simulink model "Antriebsstrangmodell_V1_4_n5"  (R2019a)
settings: Solver=FixedStepAuto  StartTime=0.0  StopTime=t_Simulation  FixedStep=dt  RelTol=1e-3
values from neighbouring files (symbols this model uses):
  A_Stirn = 2    [SIMULA~1.M]    (also in SIMULA~2.M)
  alpha_Luft = -4e-3    (= -0.004)    [SIMULA~1.M]    (also in SIMULA~2.M)
  alpha_Rotor = alpha_Al    (= 0.004)    [SIMULA~1.M]    (also in SIMULA~2.M)
  alpha_Stator = alpha_Al    (= 0.004)    [SIMULA~1.M]    (also in SIMULA~2.M)
  alpha_Ummag = -0.75e-3    (= -0.00075)    [SIMULA~1.M]    (also in SIMULA~2.M)
  c_W = 0.37    [SIMULA~1.M]    (also in SIMULA~2.M)
  COG_x = 1.4267    [SIMULA~1.M]    (also in SIMULA~2.M)
  COG_z = 0.4572    [SIMULA~1.M]    (also in SIMULA~2.M)
  cp_Luft = 1008.8    [SIMULA~1.M]    (also in SIMULA~2.M)
  e_Fahrzeug = 1.0478    [SIMULA~1.M]    (also in SIMULA~2.M)
  eta_EMaschine_Break_M_EMaschine = flipud(KennfeldMaschine.M(:,1))'    [SIMULA~1.M]    (also in SIMULA~2.M)
  eta_EMaschine_Break_M_EMaschine_reku = -KennfeldMaschine.M(:,1)'    [SIMULA~1.M]    (also in SIMULA~2.M)
  eta_EMaschine_Break_n_EMaschine = KennfeldMaschine.n(end-1,:)    [SIMULA~1.M]    (also in SIMULA~2.M)
  eta_EMaschine_Break_n_EMaschine_reku = KennfeldMaschine.n(end-1,:)    [SIMULA~1.M]    (also in SIMULA~2.M)
  eta_EMaschine_Faktor_Volllast = 0.98    [SIMULA~1.M]    (also in SIMULA~2.M)
  eta_EMaschine_Table = flip(KennfeldMaschine.etages,1)    [SIMULA~1.M]    (also in SIMULA~2.M)
  eta_EMaschine_Table_reku = KennfeldMaschine.etages    [SIMULA~1.M]    (also in SIMULA~2.M)
  eta_Getriebe = 0.96    [SIMULA~1.M]    (also in SIMULA~2.M)
  eta_IA = 0.5    [SIMULA~1.M]    (also in SIMULA~2.M)
  h_WC_pumpoff = Nu_WC*lam_WC/dh_WC    [SIMULA~1.M]    (also in SIMULA~2.M)
  h_WC_pumpon = Nu_WC*lam_WC/dh_WC    [SIMULA~1.M]    (also in SIMULA~2.M)
  i_Getriebe = 5.697    [SIMULA~1.M]    (also in SIMULA~2.M)
  krb_Korrektur = 0.53/10    (= 0.053)    [SIMULA~1.M]    (also in SIMULA~2.M)
  lam_Luft = 0.028592    [SIMULA~1.M]    (also in SIMULA~2.M)
  M_EMaschine_max = zeros(2,numel(eta_EMaschine_Break_n_EMaschine))    [SIMULA~1.M]    (also in SIMULA~2.M)
  m_Fahrzeug = 825    [SIMULA~1.M]    (also in SIMULA~2.M)
  m_Zuladung = 80    [SIMULA~1.M]    (also in SIMULA~2.M)
  nue_Luft = 19.230034390524e-6    (= 1.92300343905e-05)    [SIMULA~1.M]    (also in SIMULA~2.M)
  pump_start_limit = 273.15 + 33    (= 306.15)    [SIMULA~1.M]    (also in SIMULA~2.M)
  r_dynamisch = 0.2774    [SIMULA~1.M]    (also in SIMULA~2.M)
  rho_Luft = 1.2    [SIMULA~1.M]    (also in SIMULA~2.M)
  rho_Luft_EM = 1.0468    [SIMULA~1.M]    (also in SIMULA~2.M)
  share_EMaschine_Ummagnet_reku_Table = ser.gen.share_Ummagnetisierungsverluste    [SIMULA~1.M]    (also in SIMULA~2.M)
  share_EMaschine_Ummagnet_Table = ser.mot.share_Ummagnetisierungsverluste    [SIMULA~1.M]    (also in SIMULA~2.M)
  share_EMaschine_Wicklung_reku_Table = ser.gen.share_Wicklungsverluste    [SIMULA~1.M]    (also in SIMULA~2.M)
  share_EMaschine_Wicklung_Table = ser.mot.share_Wicklungsverluste    [SIMULA~1.M]    (also in SIMULA~2.M)
  share_EMaschine_WirkMech_reku_Table = ser.gen.share_WirkmechVerluste    [SIMULA~1.M]    (also in SIMULA~2.M)
  share_EMaschine_WirkMech_Table = ser.mot.share_WirkmechVerluste    [SIMULA~1.M]    (also in SIMULA~2.M)
  share_EMaschine_WirkZus_reku_Table = ser.gen.share_WirkZusVerl    [SIMULA~1.M]    (also in SIMULA~2.M)
  share_EMaschine_WirkZus_Table = ser.mot.share_WirkZusVerl    [SIMULA~1.M]    (also in SIMULA~2.M)
  T_Entwurf_Rotor = 273.15+20    (= 293.15)    [SIMULA~1.M]    (also in SIMULA~2.M)
  T_Entwurf_Stator = 273.15+20    (= 293.15)    [SIMULA~1.M]    (also in SIMULA~2.M)
  t_Simulation = v_Fahrzeug.Time(end)+1    [SIMULA~1.M]    (also in SIMULA~2.M = v_Fahrzeug.Time(end))
  T_Start_EMaschine = 273.15 + 23    (= 296.15)    [SIMULA~1.M]    (also in SIMULA~2.M)
  v_max = 110    [SIMULA~1.M]    (also in SIMULA~2.M)
  WB = 2.96    [SIMULA~1.M]    (also in SIMULA~2.M)
undefined symbols (not defined in the file or in its folder): A_AGP, A_IA, Anteil_Rotor_Ringe, Anteil_Stator, chi_Lager, D_2a, D_2r, delta, f_R, m_RTO, m_RYO, m_SSL_L, m_STO, m_SYO, m_WH_L, n_dis
libraries: fl_lib x440, nesl_utility x106, SimscapeCustomBlocks_lib x45, simulink x3
(part 4 of 5)

== system Antriebsstrangmodell_V1_4_n5/Antriebsstrang/E-Maschine Thermik/Wärmeübergangskoeffizienten Konvektion Luftspalt und Endcap-Luft ==
  <n_EMaschine [min^-1]> : Inport
  Abs : Abs
  Constant : Constant  Value=D_2a
  Divide : Product  Inputs=**
  Endcap-Luft-Konvektion : Subsystem
  Gain : Gain  Gain=2*pi/60
  Gain1 : Gain  Gain=0.5
  Luftspalt-Konvektion : Subsystem
  HTC_Luftspalt [W*m^-2*K^-1] : Outport
  HTC_fconv_Luftspalt [W*m^-2*K^-1] : Outport  Port=2
  HTC_Innenluft [W*m^-2*K^-1] : Outport  Port=3
  HTC_fconv_Innenluft [W*m^-2*K^-1] : Outport  Port=4
  wires:
  Gain1/1 -> Luftspalt-Konvektion/1(Rotorradius [m]), Divide/1  "Rotorradius [m]"
  <n_EMaschine [min^-1]>/1 -> Abs/1
  Constant/1 -> Gain1/1
  Abs/1 -> Gain/1, Endcap-Luft-Konvektion/1(n_EMaschine [min^-1])
  Gain/1 -> Divide/2
  Divide/1 -> Luftspalt-Konvektion/2(v_Luftspalt [m*s^-1])  "v_Luftspalt [m*s^-1]"
  Luftspalt-Konvektion/1(HTC_Luftspalt [W*m^-2*K^-1]) -> HTC_Luftspalt [W*m^-2*K^-1]/1
  Endcap-Luft-Konvektion/1(HTC_Innenluft [W*m^-2*K^-1]) -> HTC_Innenluft [W*m^-2*K^-1]/1
  Endcap-Luft-Konvektion/2(HTC_fconv_Innenluft [W*m^-2*K^-1]) -> HTC_fconv_Innenluft [W*m^-2*K^-1]/1
  Luftspalt-Konvektion/2(HTC_fconv_Luftspalt [W*m^-2*K^-1]) -> HTC_fconv_Luftspalt [W*m^-2*K^-1]/1

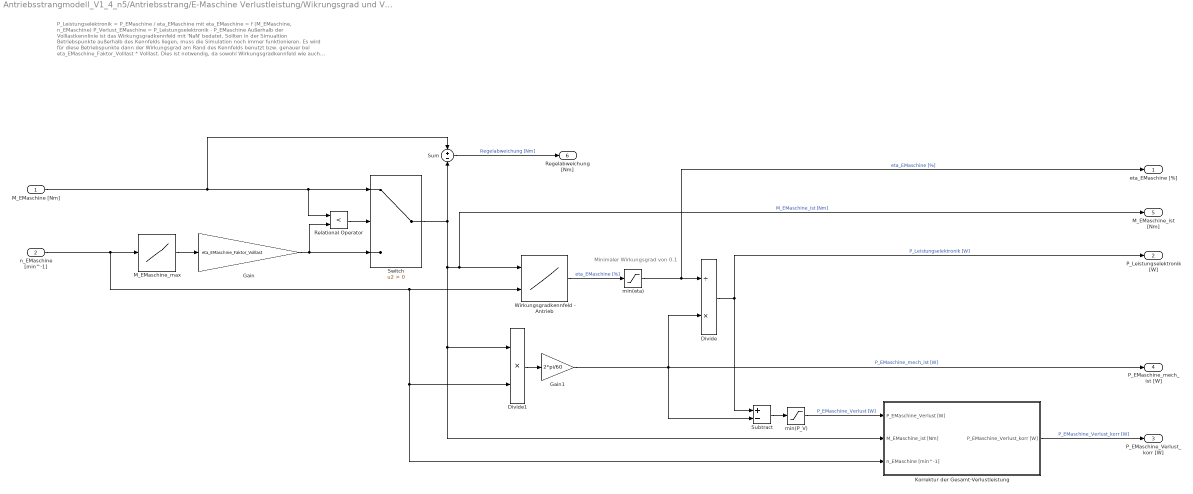
== system Antriebsstrangmodell_V1_4_n5/Antriebsstrang/E-Maschine Verlustleistung/Wikrungsgrad und Verlustleistung - Antrieb ==
  note: Minimaler Wirkungsgrad von 0.1
  note: P_Leistungselektronik = P_EMaschine / eta_EMaschine
      |
      | mit eta_EMaschine = f (M_EMaschine, n_EMaschine)
      |
      | P_Verlust_EMaschine = P_Leistungselektronik - P_EMaschine
      |
      | Außerhalb der Volllastkennlinie ist das Wirkungsgradkennfeld mit 'NaN' bedatet. Sollten in der Simualtion Betriebspunkte außerhalb des Kennfelds liegen, muss die Simulation noch immer funktionieren. Es wird für diese Betriebspunkte dann der Wirkungsgrad am Rand des Kennfelds benutzt bzw. genauer bei eta_EMaschine_Faktor_Volllast * Volllast. Dies ist notwendig, da sowohl Wirkungsgradkennfeld wie auch Lookup Table nicht stetig sind und somit zwischen Stützstellen interpolieren müssen. Dies kann dazu führen, dass ein Wert, der auf der Volllastlinie sitzt, in 'NaN' im Wirkungsgradkennfeld resultiert. Um dies zu vermeiden, wird mit eta_EMaschine_Faktor_Volllast * Volllast gerechnet, wenn Betriebspunkte außerhalb des Kennfelds liegen, um 'NaN' Wirkungsgrade zu vermeiden. eta_EMaschine_Faktor_Volllast ist stark abh. von der Güte (Abstand der Stützstellen) des Wirkungsgradkennfeldes.
  M_EMaschine [Nm] : Inport
  n_EMaschine [min^-1] : Inport  Port=2
  Divide : Product  Inputs=/*
  Divide1 : Product  Inputs=**
  Gain : Gain  Gain=eta_EMaschine_Faktor_Volllast
  Gain1 : Gain  Gain=2*pi/60
  Korrektur der Gesamt-Verlustleistung : Subsystem
  M_EMaschine_max : Lookup_n-D  NumberOfTableDimensions=1  BreakpointsForDimension1=M_EMaschine_max(1,:)  BeginIndexSearchUsingPreviousIndexResult=on  Table=M_EMaschine_max(2,:)  ExtrapMethod=Clip  UseLastTableValue=on  InternalRulePriority=Speed  RndMeth=Simplest  InputSameDT=on
  Relational Operator : RelationalOperator  Operator=<  OutDataTypeStr=boolean  RndMeth=Simplest
  Subtract : Sum  Inputs=+-
  Sum : Sum  Inputs=+-
  Switch : Switch  Criteria=u2 > Threshold
  Wirkungsgradkennfeld - Antrieb : Lookup_n-D  BreakpointsForDimension1=eta_EMaschine_Break_M_EMaschine  BreakpointsForDimension2=eta_EMaschine_Break_n_EMaschine  BeginIndexSearchUsingPreviousIndexResult=on  Table=eta_EMaschine_Table  ExtrapMethod=Clip  UseLastTableValue=on  InternalRulePriority=Speed  RndMeth=Simplest  InputSameDT=on
  min(P_V) : Saturate  UpperLimit=inf  LowerLimit=0
  min(eta) : Saturate  UpperLimit=inf  LowerLimit=0.1
  eta_EMaschine [%] : Outport
  P_Leistungselektronik [W] : Outport  Port=2
  P_EMaschine_Verlust_korr [W] : Outport  Port=3
  P_EMaschine_mech_ist [W] : Outport  Port=4
  M_EMaschine_ist [Nm] : Outport  Port=5
  Regelabweichung [Nm] : Outport  Port=6
  wires:
  Relational Operator/1 -> Switch/2
  Switch/1 -> M_EMaschine_ist [Nm]/1, Wirkungsgradkennfeld - Antrieb/1, Korrektur der Gesamt-Verlustleistung/2(M_EMaschine_ist [Nm]), Divide1/1, Sum/2  "M_EMaschine_ist [Nm]"
  Subtract/1 -> min(P_V)/1
  n_EMaschine [min^-1]/1 -> Wirkungsgradkennfeld - Antrieb/2, Korrektur der Gesamt-Verlustleistung/3(n_EMaschine [min^-1]), Divide1/2, M_EMaschine_max/1
  Wirkungsgradkennfeld - Antrieb/1 -> min(eta)/1  "eta_EMaschine [%]"
  Gain/1 -> Relational Operator/2, Switch/3
  min(eta)/1 -> eta_EMaschine [%]/1, Divide/1  "eta_EMaschine [%]"
  M_EMaschine_max/1 -> Gain/1
  M_EMaschine [Nm]/1 -> Switch/1, Relational Operator/1, Sum/1
  Divide/1 -> P_Leistungselektronik [W]/1, Subtract/1  "P_Leistungselektronik [W]"
  Divide1/1 -> Gain1/1
  Gain1/1 -> Divide/2, Subtract/2, P_EMaschine_mech_ist [W]/1  "P_EMaschine_mech_ist [W]"
  Sum/1 -> Regelabweichung [Nm]/1  "Regelabweichung [Nm]"
  min(P_V)/1 -> Korrektur der Gesamt-Verlustleistung/1(P_EMaschine_Verlust [W])  "P_EMaschine_Verlust [W]"
  Korrektur der Gesamt-Verlustleistung/1(P_EMaschine_Verlust_korr [W]) -> P_EMaschine_Verlust_korr [W]/1  "P_EMaschine_Verlust_korr [W]"

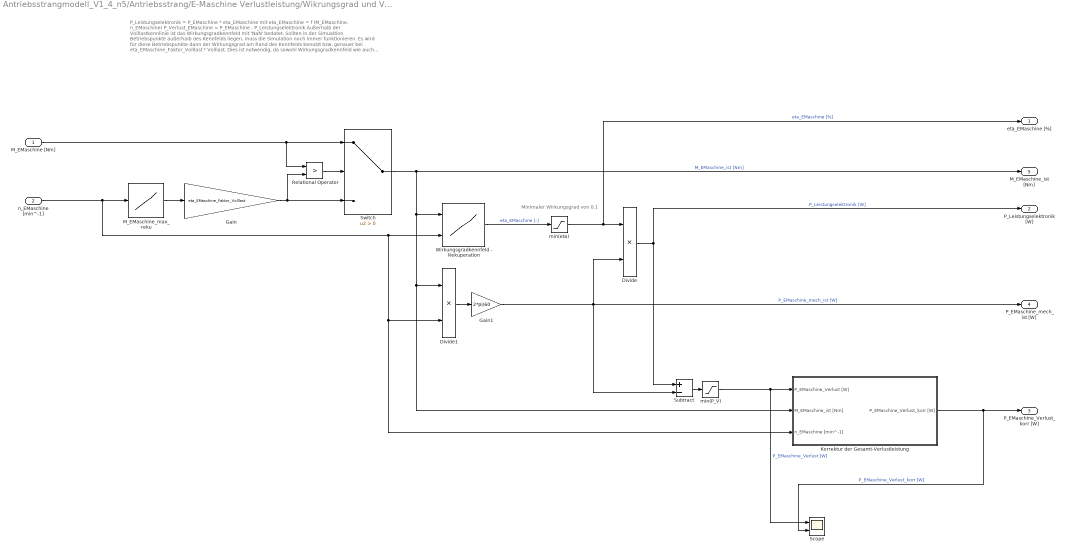
== system Antriebsstrangmodell_V1_4_n5/Antriebsstrang/E-Maschine Verlustleistung/Wikrungsgrad und Verlustleistung - Rekuperation ==
  note: Minimaler Wirkungsgrad von 0.1
  note: P_Leistungselektronik = P_EMaschine * eta_EMaschine
      |
      | mit eta_EMaschine = f (M_EMaschine, n_EMaschine)
      |
      | P_Verlust_EMaschine = P_EMaschine - P_Leistungselektronik
      |
      | Außerhalb der Volllastkennlinie ist das Wirkungsgradkennfeld mit 'NaN' bedatet. Sollten in der Simualtion Betriebspunkte außerhalb des Kennfelds liegen, muss die Simulation noch immer funktionieren. Es wird für diese Betriebspunkte dann der Wirkungsgrad am Rand des Kennfelds benutzt bzw. genauer bei eta_EMaschine_Faktor_Volllast * Volllast. Dies ist notwendig, da sowohl Wirkungsgradkennfeld wie auch Lookup Table nicht stetig sind und somit zwischen Stützstellen interpolieren müssen. Dies kann dazu führen, dass ein Wert, der auf der Volllastlinie sitzt, in 'NaN' im Wirkungsgradkennfeld resultiert. Um dies zu vermeiden, wird mit eta_EMaschine_Faktor_Volllast * Volllast gerechnet, wenn Betriebspunkte außerhalb des Kennfelds liegen, um 'NaN' Wirkungsgrade zu vermeiden. eta_EMaschine_Faktor_Volllast ist stark abh. von der Güte (Abstand der Stützstellen) des Wirkungsgradkennfeldes.
  M_EMaschine [Nm] : Inport
  n_EMaschine [min^-1] : Inport  Port=2
  Divide : Product  Inputs=**
  Divide1 : Product  Inputs=**
  Gain : Gain  Gain=eta_EMaschine_Faktor_Volllast
  Gain1 : Gain  Gain=2*pi/60
  Korrektur der Gesamt-Verlustleistung : Subsystem
  M_EMaschine_max_reku : Lookup_n-D  NumberOfTableDimensions=1  BreakpointsForDimension1=[-15,1650,2050,3400,4050,6100]  BeginIndexSearchUsingPreviousIndexResult=on  Table=[-3,-52,-50,-36.5,-32.5,-27]  ExtrapMethod=Clip  UseLastTableValue=on  InternalRulePriority=Speed  RndMeth=Simplest  InputSameDT=on
  Relational Operator : RelationalOperator  Operator=>  OutDataTypeStr=boolean  RndMeth=Simplest
  Scope : Scope  NumInputPorts=2
  Subtract : Sum  Inputs=+-
  Switch : Switch  Criteria=u2 > Threshold
  Wirkungsgradkennfeld - Rekuperation : Lookup_n-D  BreakpointsForDimension1=eta_EMaschine_Break_M_EMaschine_reku  BreakpointsForDimension2=eta_EMaschine_Break_n_EMaschine_reku  BeginIndexSearchUsingPreviousIndexResult=on  Table=eta_EMaschine_Table_reku  ExtrapMethod=Clip  UseLastTableValue=on  InternalRulePriority=Speed  RndMeth=Simplest  InputSameDT=on
  min(P_V) : Saturate  UpperLimit=inf  LowerLimit=0
  min(eta) : Saturate  UpperLimit=inf  LowerLimit=0.1
  eta_EMaschine [%] : Outport
  P_Leistungselektronik [W] : Outport  Port=2
  P_EMaschine_Verlust_korr [W] : Outport  Port=3
  P_EMaschine_mech_ist [W] : Outport  Port=4
  M_EMaschine_ist [Nm] : Outport  Port=5
  wires:
  Relational Operator/1 -> Switch/2
  Switch/1 -> Korrektur der Gesamt-Verlustleistung/2(M_EMaschine_ist [Nm]), Divide1/1, Wirkungsgradkennfeld - Rekuperation/1, M_EMaschine_ist [Nm]/1  "M_EMaschine_ist [Nm]"
  Subtract/1 -> min(P_V)/1
  n_EMaschine [min^-1]/1 -> Korrektur der Gesamt-Verlustleistung/3(n_EMaschine [min^-1]), Divide1/2, Wirkungsgradkennfeld - Rekuperation/2, M_EMaschine_max_reku/1
  Wirkungsgradkennfeld - Rekuperation/1 -> min(eta)/1  "eta_EMaschine [-]"
  Gain/1 -> Relational Operator/2, Switch/3
  min(eta)/1 -> eta_EMaschine [%]/1, Divide/1  "eta_EMaschine [%]"
  M_EMaschine_max_reku/1 -> Gain/1
  M_EMaschine [Nm]/1 -> Switch/1, Relational Operator/1
  Divide/1 -> P_Leistungselektronik [W]/1, Subtract/1  "P_Leistungselektronik [W]"
  Divide1/1 -> Gain1/1
  Gain1/1 -> Subtract/2, P_EMaschine_mech_ist [W]/1, Divide/2  "P_EMaschine_mech_ist [W]"
  min(P_V)/1 -> Scope/1, Korrektur der Gesamt-Verlustleistung/1(P_EMaschine_Verlust [W])  "P_EMaschine_Verlust [W]"
  Korrektur der Gesamt-Verlustleistung/1(P_EMaschine_Verlust_korr [W]) -> Scope/2, P_EMaschine_Verlust_korr [W]/1  "P_EMaschine_Verlust_korr [W]"

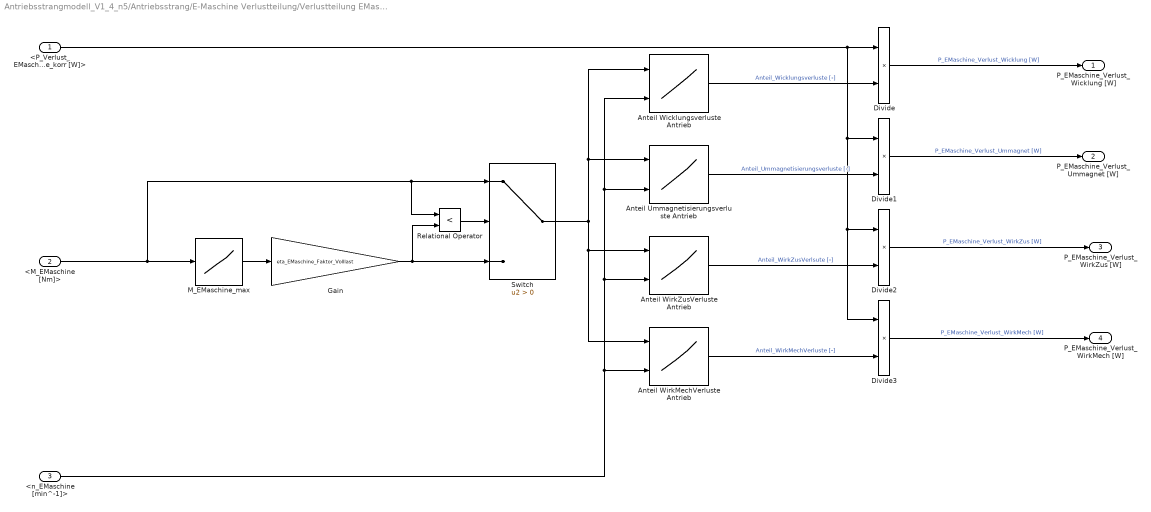
== system Antriebsstrangmodell_V1_4_n5/Antriebsstrang/E-Maschine Verlustteilung/Verlustteilung EMaschine - Antrieb ==
  <P_Verlust_EMaschine_korr [W]> : Inport
  <M_EMaschine [Nm]> : Inport  Port=2
  <n_EMaschine [min^-1]> : Inport  Port=3
  Anteil Ummagnetisierungsverluste Antrieb : Lookup_n-D  BreakpointsForDimension1=eta_EMaschine_Break_M_EMaschine  BreakpointsForDimension2=eta_EMaschine_Break_n_EMaschine  BeginIndexSearchUsingPreviousIndexResult=on  Table=share_EMaschine_Ummagnet_Table  ExtrapMethod=Clip  UseLastTableValue=on  InternalRulePriority=Speed  RndMeth=Simplest  InputSameDT=on
  Anteil Wicklungsverluste Antrieb : Lookup_n-D  BreakpointsForDimension1=eta_EMaschine_Break_M_EMaschine  BreakpointsForDimension2=eta_EMaschine_Break_n_EMaschine  BeginIndexSearchUsingPreviousIndexResult=on  Table=share_EMaschine_Wicklung_Table  ExtrapMethod=Clip  UseLastTableValue=on  InternalRulePriority=Speed  RndMeth=Simplest  InputSameDT=on
  Anteil WirkMechVerluste Antrieb : Lookup_n-D  BreakpointsForDimension1=eta_EMaschine_Break_M_EMaschine  BreakpointsForDimension2=eta_EMaschine_Break_n_EMaschine  BeginIndexSearchUsingPreviousIndexResult=on  Table=share_EMaschine_WirkMech_Table  ExtrapMethod=Clip  UseLastTableValue=on  InternalRulePriority=Speed  RndMeth=Simplest  InputSameDT=on
  Anteil WirkZusVerluste Antrieb : Lookup_n-D  BreakpointsForDimension1=eta_EMaschine_Break_M_EMaschine  BreakpointsForDimension2=eta_EMaschine_Break_n_EMaschine  BeginIndexSearchUsingPreviousIndexResult=on  Table=share_EMaschine_WirkZus_Table  ExtrapMethod=Clip  UseLastTableValue=on  InternalRulePriority=Speed  RndMeth=Simplest  InputSameDT=on
  Divide{,1..3} (4 alike) : Product  Inputs=**
  Gain : Gain  Gain=eta_EMaschine_Faktor_Volllast
  M_EMaschine_max : Lookup_n-D  NumberOfTableDimensions=1  BreakpointsForDimension1=M_EMaschine_max(1,:)  BeginIndexSearchUsingPreviousIndexResult=on  Table=M_EMaschine_max(2,:)  ExtrapMethod=Clip  UseLastTableValue=on  InternalRulePriority=Speed  RndMeth=Simplest  InputSameDT=on
  Relational Operator : RelationalOperator  Operator=<  OutDataTypeStr=boolean  RndMeth=Simplest
  Switch : Switch  Criteria=u2 > Threshold
  P_EMaschine_Verlust_Wicklung [W] : Outport
  P_EMaschine_Verlust_Ummagnet [W] : Outport  Port=2
  P_EMaschine_Verlust_WirkZus [W] : Outport  Port=3
  P_EMaschine_Verlust_WirkMech [W] : Outport  Port=4
  wires:
  Anteil Wicklungsverluste Antrieb/1 -> Divide/2  "Anteil_Wicklungsverluste [-]"
  M_EMaschine_max/1 -> Gain/1
  <n_EMaschine [min^-1]>/1 -> Anteil Wicklungsverluste Antrieb/2, Anteil Ummagnetisierungsverluste Antrieb/2, Anteil WirkZusVerluste Antrieb/2, Anteil WirkMechVerluste Antrieb/2
  <P_Verlust_EMaschine_korr [W]>/1 -> Divide3/1, Divide2/1, Divide1/1, Divide/1
  Gain/1 -> Relational Operator/2, Switch/3
  Anteil WirkMechVerluste Antrieb/1 -> Divide3/2  "Anteil_WirkMechVerluste [-]"
  Switch/1 -> Anteil WirkMechVerluste Antrieb/1, Anteil WirkZusVerluste Antrieb/1, Anteil Wicklungsverluste Antrieb/1, Anteil Ummagnetisierungsverluste Antrieb/1
  Relational Operator/1 -> Switch/2
  Divide/1 -> P_EMaschine_Verlust_Wicklung [W]/1  "P_EMaschine_Verlust_Wicklung [W]"
  Anteil Ummagnetisierungsverluste Antrieb/1 -> Divide1/2  "Anteil_Ummagnetisierungsverluste [-]"
  Anteil WirkZusVerluste Antrieb/1 -> Divide2/2  "Anteil_WirkZusVerlsute [-]"
  Divide3/1 -> P_EMaschine_Verlust_WirkMech [W]/1  "P_EMaschine_Verlust_WirkMech [W]"
  Divide1/1 -> P_EMaschine_Verlust_Ummagnet [W]/1  "P_EMaschine_Verlust_Ummagnet [W]"
  Divide2/1 -> P_EMaschine_Verlust_WirkZus [W]/1  "P_EMaschine_Verlust_WirkZus [W]"
  <M_EMaschine [Nm]>/1 -> Relational Operator/1, Switch/1, M_EMaschine_max/1

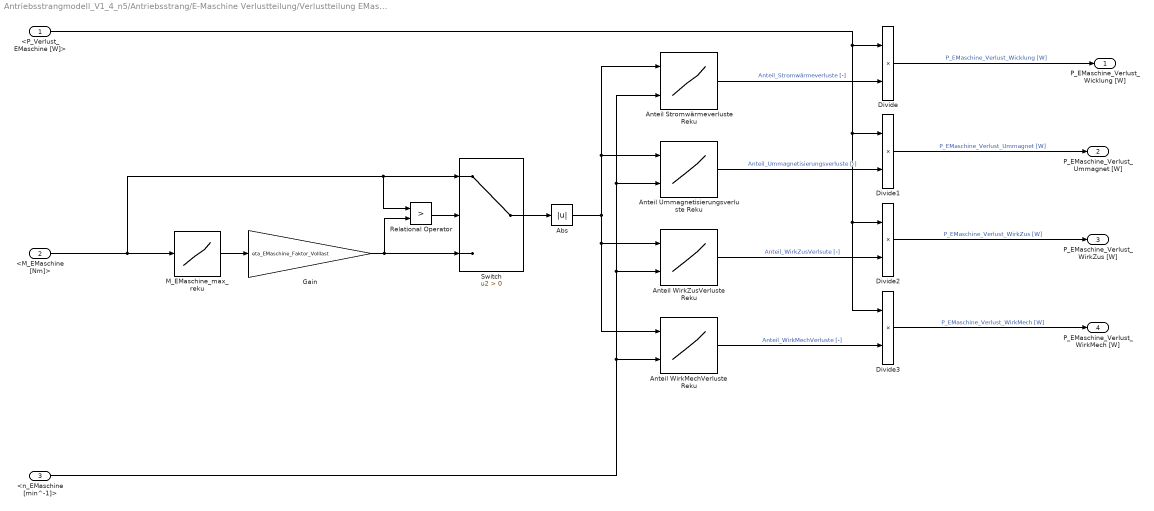
== system Antriebsstrangmodell_V1_4_n5/Antriebsstrang/E-Maschine Verlustteilung/Verlustteilung EMaschine - Rekuperation ==
  <P_Verlust_EMaschine [W]> : Inport
  <M_EMaschine [Nm]> : Inport  Port=2
  <n_EMaschine [min^-1]> : Inport  Port=3
  Abs : Abs
  Anteil Stromwärmeverluste Reku : Lookup_n-D  BreakpointsForDimension1=eta_EMaschine_Break_M_EMaschine  BreakpointsForDimension2=eta_EMaschine_Break_n_EMaschine  BeginIndexSearchUsingPreviousIndexResult=on  Table=share_EMaschine_Wicklung_reku_Table  ExtrapMethod=Clip  UseLastTableValue=on  InternalRulePriority=Speed  RndMeth=Simplest  InputSameDT=on
  Anteil Ummagnetisierungsverluste Reku : Lookup_n-D  BreakpointsForDimension1=eta_EMaschine_Break_M_EMaschine  BreakpointsForDimension2=eta_EMaschine_Break_n_EMaschine  BeginIndexSearchUsingPreviousIndexResult=on  Table=share_EMaschine_Ummagnet_reku_Table  ExtrapMethod=Clip  UseLastTableValue=on  InternalRulePriority=Speed  RndMeth=Simplest  InputSameDT=on
  Anteil WirkMechVerluste Reku : Lookup_n-D  BreakpointsForDimension1=eta_EMaschine_Break_M_EMaschine  BreakpointsForDimension2=eta_EMaschine_Break_n_EMaschine  BeginIndexSearchUsingPreviousIndexResult=on  Table=share_EMaschine_WirkMech_reku_Table  ExtrapMethod=Clip  UseLastTableValue=on  InternalRulePriority=Speed  RndMeth=Simplest  InputSameDT=on
  Anteil WirkZusVerluste Reku : Lookup_n-D  BreakpointsForDimension1=eta_EMaschine_Break_M_EMaschine  BreakpointsForDimension2=eta_EMaschine_Break_n_EMaschine  BeginIndexSearchUsingPreviousIndexResult=on  Table=share_EMaschine_WirkZus_reku_Table  ExtrapMethod=Clip  UseLastTableValue=on  InternalRulePriority=Speed  RndMeth=Simplest  InputSameDT=on
  Divide{,1..3} (4 alike) : Product  Inputs=**
  Gain : Gain  Gain=eta_EMaschine_Faktor_Volllast
  M_EMaschine_max_reku : Lookup_n-D  NumberOfTableDimensions=1  BreakpointsForDimension1=[-15,1700,2050,3400,4050,6100]  BeginIndexSearchUsingPreviousIndexResult=on  Table=[0.44,-52,-51,-37.5,-33,-27.25]  ExtrapMethod=Clip  UseLastTableValue=on  InternalRulePriority=Speed  RndMeth=Simplest  InputSameDT=on
  Relational Operator : RelationalOperator  Operator=>  OutDataTypeStr=boolean  RndMeth=Simplest
  Switch : Switch  Criteria=u2 > Threshold
  P_EMaschine_Verlust_Wicklung [W] : Outport
  P_EMaschine_Verlust_Ummagnet [W] : Outport  Port=2
  P_EMaschine_Verlust_WirkZus [W] : Outport  Port=3
  P_EMaschine_Verlust_WirkMech [W] : Outport  Port=4
  wires:
  Anteil Stromwärmeverluste Reku/1 -> Divide/2  "Anteil_Stromwärmeverluste [-]"
  M_EMaschine_max_reku/1 -> Gain/1
  <n_EMaschine [min^-1]>/1 -> Anteil Stromwärmeverluste Reku/2, Anteil Ummagnetisierungsverluste Reku/2, Anteil WirkZusVerluste Reku/2, Anteil WirkMechVerluste Reku/2
  <P_Verlust_EMaschine [W]>/1 -> Divide3/1, Divide2/1, Divide1/1, Divide/1
  Gain/1 -> Relational Operator/2, Switch/3
  Anteil WirkMechVerluste Reku/1 -> Divide3/2  "Anteil_WirkMechVerluste [-]"
  Switch/1 -> Abs/1
  Relational Operator/1 -> Switch/2
  Divide/1 -> P_EMaschine_Verlust_Wicklung [W]/1  "P_EMaschine_Verlust_Wicklung [W]"
  Anteil Ummagnetisierungsverluste Reku/1 -> Divide1/2  "Anteil_Ummagnetisierungsverluste [-]"
  Anteil WirkZusVerluste Reku/1 -> Divide2/2  "Anteil_WirkZusVerlsute [-]"
  Divide3/1 -> P_EMaschine_Verlust_WirkMech [W]/1  "P_EMaschine_Verlust_WirkMech [W]"
  Divide1/1 -> P_EMaschine_Verlust_Ummagnet [W]/1  "P_EMaschine_Verlust_Ummagnet [W]"
  Divide2/1 -> P_EMaschine_Verlust_WirkZus [W]/1  "P_EMaschine_Verlust_WirkZus [W]"
  <M_EMaschine [Nm]>/1 -> M_EMaschine_max_reku/1, Relational Operator/1, Switch/1
  Abs/1 -> Anteil WirkMechVerluste Reku/1, Anteil WirkZusVerluste Reku/1, Anteil Stromwärmeverluste Reku/1, Anteil Ummagnetisierungsverluste Reku/1

== system Antriebsstrangmodell_V1_4_n5/Antriebsstrang/Getriebe/Antreiben ==
  note: n_EMaschine = n_Rad * i_Getriebe
      |
      | M_EMaschine = M_Rad / (i_Getriebe * eta_Getriebe)
      |
      | P_EMaschine = P_Rad / eta_Getriebe
      |
      | P_Verlust_Getriebe = P_EMaschine - P_Rad
  n_Rad [min^-1] : Inport
  M_Rad [Nm] : Inport  Port=2
  P_Rad [W] : Inport  Port=3
  Constant : Constant  Value=i_Getriebe
  Constant1 : Constant  Value=eta_Getriebe
  Divide : Product  Inputs=/*/
  Divide1 : Product  Inputs=/*
  Product : Product
  Subtract : Sum  Inputs=+-
  n_EMaschine [min^-1] : Outport
  M_EMaschine [Nm] : Outport  Port=2
  P_EMaschine [W] : Outport  Port=3
  P_Verlust_Getriebe [W] : Outport  Port=4
  wires:
  Divide1/1 -> P_EMaschine [W]/1, Subtract/1  "P_EMaschine [W]"
  Constant1/1 -> Divide1/1, Divide/3
  Constant/1 -> Divide/1, Product/2
  Product/1 -> n_EMaschine [min^-1]/1  "n_EMaschine [min^-1]"
  P_Rad [W]/1 -> Subtract/2, Divide1/2
  M_Rad [Nm]/1 -> Divide/2
  Divide/1 -> M_EMaschine [Nm]/1  "M_EMaschine [Nm]"
  n_Rad [min^-1]/1 -> Product/1
  Subtract/1 -> P_Verlust_Getriebe [W]/1  "P_Verlust_Getriebe [W]"

== system Antriebsstrangmodell_V1_4_n5/Antriebsstrang/Getriebe/Rekuperieren ==
  note: n_EMaschine = n_Rad * i_Getriebe
      |
      | M_EMaschine = M_Rad * eta_Getriebe / i_Getriebe
      |
      | P_EMaschine = P_Rad * eta_Getriebe
      |
      | P_Verlust_Getriebe = P_EMaschine - P_Rad
  n_Rad [min^-1] : Inport
  M_Rad [Nm] : Inport  Port=2
  P_Rad [W] : Inport  Port=3
  Constant : Constant  Value=i_Getriebe
  Constant1 : Constant  Value=eta_Getriebe
  Divide : Product  Inputs=/**
  Divide1 : Product  Inputs=**
  Product : Product
  Subtract : Sum  Inputs=+-
  n_EMaschine [min^-1] : Outport
  M_EMaschine [Nm] : Outport  Port=2
  P_EMaschine [W] : Outport  Port=3
  P_Verlust_Getriebe [W] : Outport  Port=4
  wires:
  Divide1/1 -> P_EMaschine [W]/1, Subtract/1  "P_EMaschine [W]"
  Constant1/1 -> Divide1/1, Divide/3
  Constant/1 -> Divide/1, Product/2
  Product/1 -> n_EMaschine [min^-1]/1  "n_EMaschine [min^-1]"
  P_Rad [W]/1 -> Subtract/2, Divide1/2
  M_Rad [Nm]/1 -> Divide/2
  Divide/1 -> M_EMaschine [Nm]/1  "M_EMaschine [Nm]"
  n_Rad [min^-1]/1 -> Product/1
  Subtract/1 -> P_Verlust_Getriebe [W]/1  "P_Verlust_Getriebe [W]"

== system Antriebsstrangmodell_V1_4_n5/Antriebsstrang/Rad/Dynamische Antriebsleistungsverteilung Allradbetrieb ==
  note: X_HA,Achslast = (COG_x + a_Fahrzeug/9.81*COG_z) / WB
  M_Raeder [Nm] : Inport
  a_Fahrzeug [m*s^-2] : Inport  Port=2
  Add : Sum
  Constant : Constant  Value=COG_x
  Constant1 : Constant  Value=COG_z
  Constant2 : Constant  Value=WB
  Constant7 : Constant  Value=9.81  VectorParams1D=off
  Divide : Product  Inputs=*/
  Divide1 : Product  Inputs=**
  Divide2 : Product  Inputs=*/
  Product7 : Product
  Sum : Sum  Inputs=-+|
  M_Rad_VA [Nm] : Outport
  M_Rad_HA [Nm] : Outport  Port=2
  wires:
  Product7/1 -> Sum/1, M_Rad_HA [Nm]/1  "M_Rad_HA [Nm]"
  Constant7/1 -> Divide/2
  a_Fahrzeug [m*s^-2]/1 -> Divide/1  "a_Fahrzeug [m*s^-2]"
  Divide/1 -> Divide1/1
  Constant1/1 -> Divide1/2
  Divide1/1 -> Add/1
  Constant/1 -> Add/2
  Add/1 -> Divide2/1
  Constant2/1 -> Divide2/2
  Divide2/1 -> Product7/1  "X_HA,Achslast [-]"
  M_Raeder [Nm]/1 -> Sum/2, Product7/2
  Sum/1 -> M_Rad_VA [Nm]/1

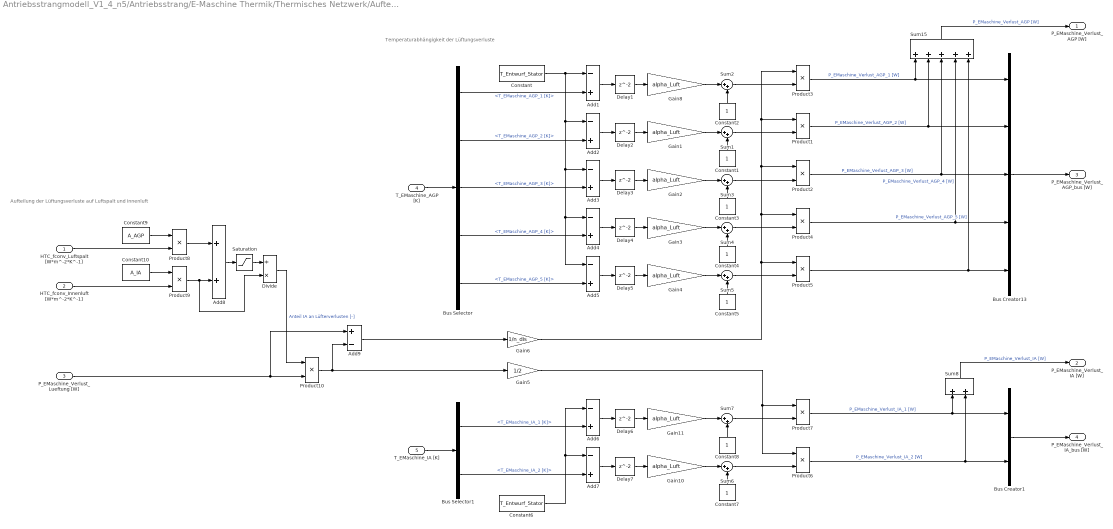
== system Antriebsstrangmodell_V1_4_n5/Antriebsstrang/E-Maschine Thermik/Thermisches Netzwerk/Aufteilung + Temperaturabhängigkeit Lüftungsverluste ==
  note: Temperaturabhängigkeit der Lüftungsverluste
  note: Aufteilung der Lüftungsverluste auf Luftspalt und Innenluft
  HTC_fconv_Luftspalt [W*m^-2*K^-1] : Inport
  HTC_fconv_Innenluft [W*m^-2*K^-1] : Inport  Port=2
  P_EMaschine_Verlust_Lueftung [W] : Inport  Port=3
  T_EMaschine_AGP [K] : Inport  Port=4
  T_EMaschine_IA [K] : Inport  Port=5
  Add{1..7} (7 alike) : Sum  Inputs=-+
  Add8 : Sum
  Add9 : Sum  Inputs=+-
  Bus Creator1 : BusCreator  Inputs=2
  Bus Creator13 : BusCreator  Inputs=5
  Bus Selector : BusSelector  OutputSignals=T_EMaschine_AGP_1 [K],T_EMaschine_AGP_2 [K],T_EMaschine_AGP_3 [K],T_EMaschine_AGP_4 [K],T_EMaschine_AGP_5 [K]
  Bus Selector1 : BusSelector  OutputSignals=T_EMaschine_IA_1 [K],T_EMaschine_IA_2 [K]
  Constant : Constant  Value=T_Entwurf_Stator
  Constant{1..5,7..8} (7 alike) : Constant
  Constant10 : Constant  Value=A_IA
  Constant6 : Constant  Value=T_Entwurf_Stator
  Constant9 : Constant  Value=A_AGP
  Delay{1..7} (7 alike) : Delay
  Divide : Product  Inputs=/*
  Gain{1..4,8,10..11} (7 alike) : Gain  Gain=alpha_Luft
  Gain5 : Gain  Gain=1/2
  Gain6 : Gain  Gain=1/n_dis
  Product{1..10} (10 alike) : Product
  Saturation : Saturate  UpperLimit=1e6  LowerLimit=0.001
  Sum{1..7} (7 alike) : Sum  Inputs=|++
  Sum15 : Sum  Inputs=+++++
  Sum8 : Sum
  P_EMaschine_Verlust_AGP [W] : Outport
  P_EMaschine_Verlust_IA [W] : Outport  Port=2
  P_EMaschine_Verlust_AGP_bus [W] : Outport  Port=3
  P_EMaschine_Verlust_IA_bus [W] : Outport  Port=4
  wires:
  Sum2/1 -> Product3/2
  Gain8/1 -> Sum2/1
  Delay1/1 -> Gain8/1
  Add1/1 -> Delay1/1
  Constant2/1 -> Sum2/2
  T_EMaschine_AGP [K]/1 -> Bus Selector/1
  Delay2/1 -> Gain1/1
  Add2/1 -> Delay2/1
  Constant1/1 -> Sum1/2
  Sum1/1 -> Product1/2
  Gain1/1 -> Sum1/1
  Gain2/1 -> Sum3/1
  Sum3/1 -> Product2/2
  Add3/1 -> Delay3/1
  Constant3/1 -> Sum3/2
  Delay3/1 -> Gain2/1
  Gain3/1 -> Sum4/1
  Sum4/1 -> Product4/2
  Add4/1 -> Delay4/1
  Constant4/1 -> Sum4/2
  Delay4/1 -> Gain3/1
  Gain4/1 -> Sum5/1
  Constant/1 -> Add3/1, Add5/1, Add4/1, Add2/1, Add1/1
  Sum5/1 -> Product5/2
  Add5/1 -> Delay5/1
  Constant5/1 -> Sum5/2
  Delay5/1 -> Gain4/1
  Bus Selector/1 -> Add1/2  "<T_EMaschine_AGP_1 [K]>"
  Bus Selector/2 -> Add2/2  "<T_EMaschine_AGP_2 [K]>"
  Bus Selector/3 -> Add3/2  "<T_EMaschine_AGP_3 [K]>"
  Bus Selector/4 -> Add4/2  "<T_EMaschine_AGP_4 [K]>"
  Bus Selector/5 -> Add5/2  "<T_EMaschine_AGP_5 [K]>"
  Product2/1 -> Bus Creator13/3, Sum15/3  "P_EMaschine_Verlust_AGP_3 [W]"
  Product4/1 -> Bus Creator13/4, Sum15/4  "P_EMaschine_Verlust_AGP_4 [W]"
  Product5/1 -> Sum15/5, Bus Creator13/5  "P_EMaschine_Verlust_AGP_5 [W]"
  Gain6/1 -> Product3/1, Product1/1, Product2/1, Product4/1, Product5/1
  Product1/1 -> Sum15/2, Bus Creator13/2  "P_EMaschine_Verlust_AGP_2 [W]"
  Product3/1 -> Bus Creator13/1, Sum15/1  "P_EMaschine_Verlust_AGP_1 [W]"
  Bus Creator13/1 -> P_EMaschine_Verlust_AGP_bus [W]/1
  Sum15/1 -> P_EMaschine_Verlust_AGP [W]/1  "P_EMaschine_Verlust_AGP [W]"
  Product10/1 -> Gain5/1, Add9/2
  T_EMaschine_IA [K]/1 -> Bus Selector1/1
  Sum6/1 -> Product6/2
  Constant6/1 -> Add6/1, Add7/1
  Add7/1 -> Delay7/1
  Delay7/1 -> Gain10/1
  Constant8/1 -> Sum7/2
  Sum7/1 -> Product7/2
  Bus Selector1/2 -> Add7/2  "<T_EMaschine_IA_2 [K]>"
  Product7/1 -> Sum8/1, Bus Creator1/1  "P_EMaschine_Verlust_IA_1 [W]"
  Gain11/1 -> Sum7/1
  Bus Selector1/1 -> Add6/2  "<T_EMaschine_IA_1 [K]>"
  Constant7/1 -> Sum6/2
  Delay6/1 -> Gain11/1
  Gain10/1 -> Sum6/1
  Add6/1 -> Delay6/1
  Product6/1 -> Sum8/2, Bus Creator1/2  "P_EMaschine_Verlust_IA_2 [W]"
  Gain5/1 -> Product6/1, Product7/1
  Sum8/1 -> P_EMaschine_Verlust_IA [W]/1  "P_EMaschine_Verlust_IA [W]"
  Bus Creator1/1 -> P_EMaschine_Verlust_IA_bus [W]/1
  HTC_fconv_Luftspalt [W*m^-2*K^-1]/1 -> Product8/2
  Constant9/1 -> Product8/1
  Constant10/1 -> Product9/1
  Product8/1 -> Add8/1
  Product9/1 -> Divide/2, Add8/2
  Add8/1 -> Saturation/1
  P_EMaschine_Verlust_Lueftung [W]/1 -> Product10/2, Add9/1
  Divide/1 -> Product10/1  "Anteil IA an Lüfterverlusten [-]"
  HTC_fconv_Innenluft [W*m^-2*K^-1]/1 -> Product9/2
  Saturation/1 -> Divide/1
  Add9/1 -> Gain6/1

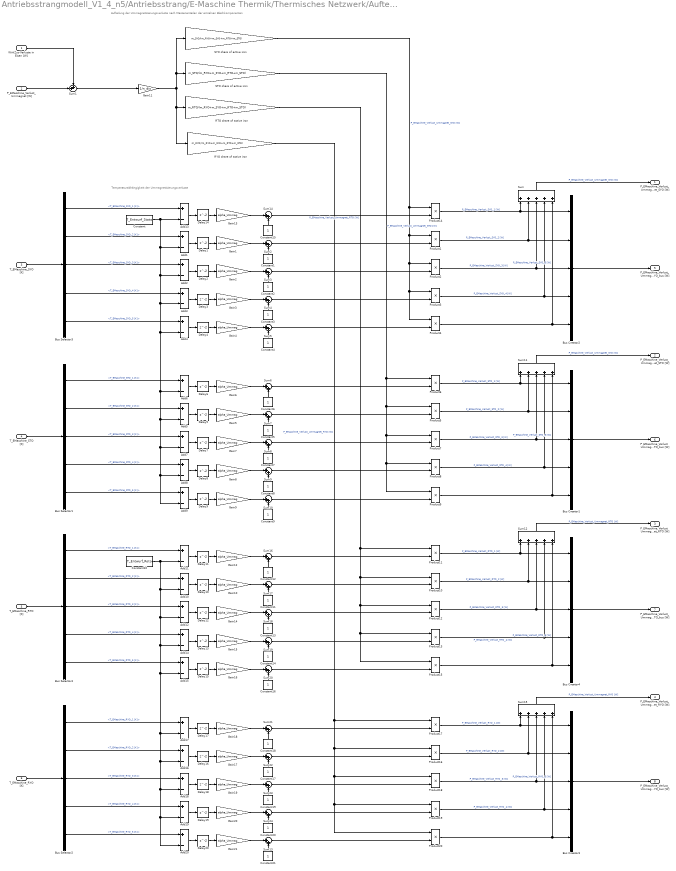
== system Antriebsstrangmodell_V1_4_n5/Antriebsstrang/E-Maschine Thermik/Thermisches Netzwerk/Aufteilung + Temperaturabhängigkeit Ummagnetisierungsverluste ==
  note: Temperaturabhängigkeit der Ummagnetisierungsverluste
  note: Aufteilung der Ummagnetisierungsverluste nach Massenanteilen der einzelnen Blechkomponenten
  WirkZus-Verluste in Eisen [W] : Inport
  P_EMaschine_Verlust_Ummagnet [W] : Inport  Port=2
  T_EMaschine_SYO [K] : Inport  Port=3
  T_EMaschine_STO [K] : Inport  Port=4
  T_EMaschine_RTO [K] : Inport  Port=5
  T_EMaschine_RYO [K] : Inport  Port=6
  Add{1..20} (20 alike) : Sum  Inputs=+-
  Bus Creator{1..4} (4 alike) : BusCreator  Inputs=5
  Bus Selector1 : BusSelector  OutputSignals=T_EMaschine_STO_1 [K],T_EMaschine_STO_2 [K],T_EMaschine_STO_3 [K],T_EMaschine_STO_4 [K],T_EMaschine_STO_5 [K]
  Bus Selector2 : BusSelector  OutputSignals=T_EMaschine_RYO_1 [K],T_EMaschine_RYO_2 [K],T_EMaschine_RYO_3 [K],T_EMaschine_RYO_4 [K],T_EMaschine_RYO_5 [K]
  Bus Selector3 : BusSelector  OutputSignals=T_EMaschine_SYO_1 [K],T_EMaschine_SYO_2 [K],T_EMaschine_SYO_3 [K],T_EMaschine_SYO_4 [K],T_EMaschine_SYO_5 [K]
  Bus Selector4 : BusSelector  OutputSignals=T_EMaschine_RTO_1 [K],T_EMaschine_RTO_2 [K],T_EMaschine_RTO_3 [K],T_EMaschine_RTO_4 [K],T_EMaschine_RTO_5 [K]
  Constant : Constant  Value=T_Entwurf_Stator
  Constant{1..9,11..21} (20 alike) : Constant
  Constant10 : Constant  Value=T_Entwurf_Rotor
  Delay{1..20} (20 alike) : Delay
  Gain{1..10,12..21} (20 alike) : Gain  Gain=alpha_Ummag
  Gain11 : Gain  Gain=1/n_dis
  Product{1..20} (20 alike) : Product
  RTO share of active iron : Gain  Gain=m_RTO/(m_RYO+m_SYO+m_RTO+m_STO)
  RYO share of active iron : Gain  Gain=m_RYO/(m_RYO+m_SYO+m_RTO+m_STO)
  STO share of active iron : Gain  Gain=m_STO/(m_RYO+m_SYO+m_RTO+m_STO)
  SYO share of active iron : Gain  Gain=m_SYO/(m_RYO+m_SYO+m_RTO+m_STO)
  Sum{,11..12,15} (4 alike) : Sum  Inputs=+++++
  Sum1 : Sum  Inputs=++|
  Sum{2..10,13..14,16..24} (20 alike) : Sum  Inputs=|++
  P_EMaschine_Verlust_Ummagnet_SYO [W] : Outport
  P_EMaschine_Verlust_Ummagnet_STO [W] : Outport  Port=2
  P_EMaschine_Verlust_Ummagnet_RTO [W] : Outport  Port=3
  P_EMaschine_Verlust_Ummagnet_RYO [W] : Outport  Port=4
  P_EMaschine_Verlust_Ummagnet_SYO_bus [W] : Outport  Port=5
  P_EMaschine_Verlust_Ummagnet_STO_bus [W] : Outport  Port=6
  P_EMaschine_Verlust_Ummagnet_RTO_bus [W] : Outport  Port=7
  P_EMaschine_Verlust_Ummagnet_RYO_bus [W] : Outport  Port=8
  wires:
  P_EMaschine_Verlust_Ummagnet [W]/1 -> Sum1/2
  Sum1/1 -> Gain11/1
  WirkZus-Verluste in Eisen [W]/1 -> Sum1/1
  Sum14/1 -> Product14/2
  Product14/1 -> Sum/1, Bus Creator2/1  "P_EMaschine_Verlust_SYO_1 [W]"
  Gain13/1 -> Sum14/1
  Delay14/1 -> Gain13/1
  Add13/1 -> Delay14/1
  Constant15/1 -> Sum14/2
  Gain1/1 -> Sum2/1
  Product1/1 -> Sum/2, Bus Creator2/2  "P_EMaschine_Verlust_SYO_2 [W]"
  Add1/1 -> Delay1/1
  Constant1/1 -> Sum2/2
  Sum2/1 -> Product1/2
  Delay1/1 -> Gain1/1
  Sum3/1 -> Product2/2
  Delay2/1 -> Gain2/1
  Product2/1 -> Sum/3, Bus Creator2/3  "P_EMaschine_Verlust_SYO_3 [W]"
  Gain2/1 -> Sum3/1
  Constant2/1 -> Sum3/2
  Add2/1 -> Delay2/1
  Sum4/1 -> Product3/2
  Delay3/1 -> Gain3/1
  Product3/1 -> Bus Creator2/4, Sum/4  "P_EMaschine_Verlust_SYO_4 [W]"
  Gain3/1 -> Sum4/1
  Constant3/1 -> Sum4/2
  Add3/1 -> Delay3/1
  Sum5/1 -> Product4/2
  Delay4/1 -> Gain4/1
  Product4/1 -> Bus Creator2/5, Sum/5  "P_EMaschine_Verlust_SYO_5 [W]"
  Gain4/1 -> Sum5/1
  Constant4/1 -> Sum5/2
  Add4/1 -> Delay4/1
  Delay5/1 -> Gain5/1
  Add8/1 -> Delay8/1
  Constant8/1 -> Sum9/2
  Gain8/1 -> Sum9/1
  Sum9/1 -> Product8/2
  Product8/1 -> Sum11/4, Bus Creator1/4  "P_EMaschine_Verlust_STO_4 [W]"
  Delay8/1 -> Gain8/1
  Delay6/1 -> Gain6/1
  Constant6/1 -> Sum6/2
  Gain6/1 -> Sum6/1
  Sum7/1 -> Product5/2
  Product6/1 -> Sum11/1, Bus Creator1/1  "P_EMaschine_Verlust_STO_1 [W]"
  Sum6/1 -> Product6/2
  Add9/1 -> Delay9/1
  Add5/1 -> Delay5/1
  Product5/1 -> Sum11/2, Bus Creator1/2  "P_EMaschine_Verlust_STO_2 [W]"
  Gain5/1 -> Sum7/1
  Add7/1 -> Delay7/1
  Constant7/1 -> Sum8/2
  Delay7/1 -> Gain7/1
  Constant5/1 -> Sum7/2
  Constant/1 -> Add9/2, Add8/2, Add7/2, Add5/2, Add6/2, Add4/2, Add3/2, Add2/2, Add1/2, Add13/2
  Add6/1 -> Delay6/1
  Constant9/1 -> Sum10/2
  Sum8/1 -> Product7/2
  Gain9/1 -> Sum10/1
  Product9/1 -> Bus Creator1/5, Sum11/5  "P_EMaschine_Verlust_STO_5 [W]"
  Delay9/1 -> Gain9/1
  Gain7/1 -> Sum8/1
  Sum10/1 -> Product9/2
  Product7/1 -> Sum11/3, Bus Creator1/3  "P_EMaschine_Verlust_STO_3 [W]"
  SYO share of active iron/1 -> Product4/1, Product3/1, Product2/1, Product1/1, Product14/1  "P_EMaschine_Verlust_Ummagnet_SYO [W]"
  STO share of active iron/1 -> Product9/1, Product8/1, Product7/1, Product5/1, Product6/1  "P_EMaschine_Verlust_Ummagnet_STO [W]"
  Gain11/1 -> RYO share of active iron/1, RTO share of active iron/1, STO share of active iron/1, SYO share of active iron/1
  Sum/1 -> P_EMaschine_Verlust_Ummagnet_SYO [W]/1  "P_EMaschine_Verlust_Ummagnet_SYO [W]"
  Sum11/1 -> P_EMaschine_Verlust_Ummagnet_STO [W]/1  "P_EMaschine_Verlust_Ummagnet_SYO [W]"
  T_EMaschine_SYO [K]/1 -> Bus Selector3/1
  Bus Selector3/1 -> Add13/1  "<T_EMaschine_SYO_1 [K]>"
  Bus Selector3/2 -> Add1/1  "<T_EMaschine_SYO_2 [K]>"
  Bus Selector3/3 -> Add2/1  "<T_EMaschine_SYO_3 [K]>"
  Bus Selector3/4 -> Add3/1  "<T_EMaschine_SYO_4 [K]>"
  Bus Selector3/5 -> Add4/1  "<T_EMaschine_SYO_5 [K]>"
  Bus Selector1/4 -> Add8/1  "<T_EMaschine_STO_4 [K]>"
  Bus Selector1/2 -> Add5/1  "<T_EMaschine_STO_2 [K]>"
  Bus Selector1/3 -> Add7/1  "<T_EMaschine_STO_3 [K]>"
  Bus Selector1/5 -> Add9/1  "<T_EMaschine_STO_5 [K]>"
  T_EMaschine_STO [K]/1 -> Bus Selector1/1
  Bus Selector1/1 -> Add6/1  "<T_EMaschine_STO_1 [K]>"
  Bus Creator2/1 -> P_EMaschine_Verlust_Ummagnet_SYO_bus [W]/1
  Bus Creator1/1 -> P_EMaschine_Verlust_Ummagnet_STO_bus [W]/1
  Bus Selector4/3 -> Add12/1  "<T_EMaschine_RTO_3 [K]>"
  Delay10/1 -> Gain10/1
  Bus Creator4/1 -> P_EMaschine_Verlust_Ummagnet_RTO_bus [W]/1
  T_EMaschine_RYO [K]/1 -> Bus Selector2/1
  Bus Selector4/4 -> Add14/1  "<T_EMaschine_RTO_4 [K]>"
  Product10/1 -> Sum12/2, Bus Creator4/2  "P_EMaschine_Verlust_RTO_2 [W]"
  Bus Selector4/5 -> Add15/1  "<T_EMaschine_RTO_5 [K]>"
  Bus Selector4/2 -> Add10/1  "<T_EMaschine_RTO_2 [K]>"
  T_EMaschine_RTO [K]/1 -> Bus Selector4/1
  Product19/1 -> Sum15/4, Bus Creator3/4  "P_EMaschine_Verlust_RYO_4 [W]"
  Product11/1 -> Sum12/1, Bus Creator4/1  "P_EMaschine_Verlust_RTO_1 [W]"
  Add14/1 -> Delay13/1
  Constant14/1 -> Sum19/2
  Gain15/1 -> Sum19/1
  Sum19/1 -> Product13/2
  Delay13/1 -> Gain15/1
  Product17/1 -> Sum15/1, Bus Creator3/1  "P_EMaschine_Verlust_RYO_1 [W]"
  Sum12/1 -> P_EMaschine_Verlust_Ummagnet_RTO [W]/1  "P_EMaschine_Verlust_Ummagnet_RTO [W]"
  Product15/1 -> Bus Creator4/5, Sum12/5  "P_EMaschine_Verlust_RTO_5 [W]"
  Product13/1 -> Bus Creator4/4, Sum12/4  "P_EMaschine_Verlust_RTO_4 [W]"
  Sum15/1 -> P_EMaschine_Verlust_Ummagnet_RYO [W]/1  "P_EMaschine_Verlust_Ummagnet_RYO [W]"
  Bus Selector2/5 -> Add20/1  "<T_EMaschine_RYO_5 [K]>"
  Bus Selector2/3 -> Add18/1  "<T_EMaschine_RYO_3 [K]>"
  Bus Selector2/4 -> Add19/1  "<T_EMaschine_RYO_4 [K]>"
  Bus Selector2/2 -> Add16/1  "<T_EMaschine_RYO_2 [K]>"
  Product18/1 -> Sum15/3, Bus Creator3/3  "P_EMaschine_Verlust_RYO_3 [W]"
  Product16/1 -> Sum15/2, Bus Creator3/2  "P_EMaschine_Verlust_RYO_2 [W]"
  Constant10/1 -> Add20/2, Add19/2, Add18/2, Add16/2, Add17/2, Add15/2, Add14/2, Add12/2, Add10/2, Add11/2
  Sum17/1 -> Product10/2
  Delay11/1 -> Gain12/1
  Constant12/1 -> Sum16/2
  Add11/1 -> Delay11/1
  Gain12/1 -> Sum16/1
  Sum16/1 -> Product11/2
  Bus Selector4/1 -> Add11/1  "<T_EMaschine_RTO_1 [K]>"
  Product12/1 -> Sum12/3, Bus Creator4/3  "P_EMaschine_Verlust_RTO_3 [W]"
  Add15/1 -> Delay15/1
  Gain10/1 -> Sum17/1
  Sum24/1 -> Product19/2
  Delay19/1 -> Gain20/1
  Constant18/1 -> Sum21/2
  Delay17/1 -> Gain18/1
  Constant20/1 -> Sum24/2
  Delay16/1 -> Gain17/1
  Add19/1 -> Delay19/1
  Sum18/1 -> Product12/2
  Add10/1 -> Delay10/1
  Gain20/1 -> Sum24/1
  Gain17/1 -> Sum22/1
  Sum22/1 -> Product16/2
  Add12/1 -> Delay12/1
  Sum21/1 -> Product17/2
  Add16/1 -> Delay16/1
  Constant13/1 -> Sum18/2
  Gain18/1 -> Sum21/1
  Gain21/1 -> Sum13/1
  Constant17/1 -> Sum22/2
  Bus Selector2/1 -> Add17/1  "<T_EMaschine_RYO_1 [K]>"
  Add17/1 -> Delay17/1
  Constant21/1 -> Sum13/2
  Constant19/1 -> Sum23/2
  Delay12/1 -> Gain14/1
  Constant11/1 -> Sum17/2
  Delay18/1 -> Gain19/1
  Sum13/1 -> Product20/2
  Gain19/1 -> Sum23/1
  Bus Creator3/1 -> P_EMaschine_Verlust_Ummagnet_RYO_bus [W]/1
  Add20/1 -> Delay20/1
  Delay20/1 -> Gain21/1
  Add18/1 -> Delay18/1
  Gain16/1 -> Sum20/1
  Delay15/1 -> Gain16/1
  Sum20/1 -> Product15/2
  Gain14/1 -> Sum18/1
  Product20/1 -> Bus Creator3/5, Sum15/5  "P_EMaschine_Verlust_RYO_5 [W]"
  Constant16/1 -> Sum20/2
  Sum23/1 -> Product18/2
  RTO share of active iron/1 -> Product15/1, Product13/1, Product12/1, Product10/1, Product11/1  "P_EMaschine_Verlust_Ummagnet_RTO [W]"
  RYO share of active iron/1 -> Product17/1, Product20/1, Product19/1, Product18/1, Product16/1  "P_EMaschine_Verlust_Ummagnet_RYO [W]"

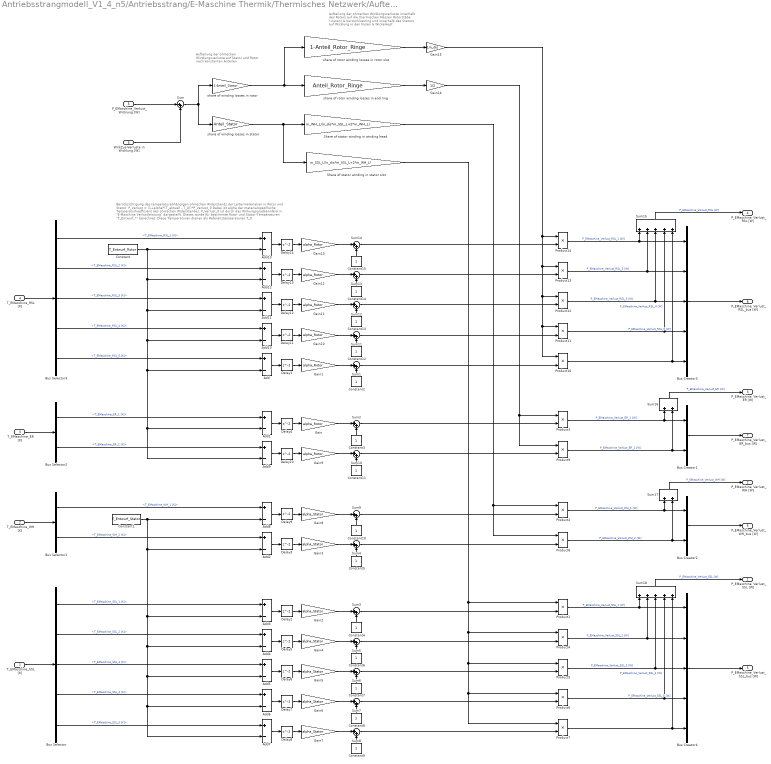
== system Antriebsstrangmodell_V1_4_n5/Antriebsstrang/E-Maschine Thermik/Thermisches Netzwerk/Aufteilung Wicklungsverluste + Temperaturabhängiger ohmscher Widerstand ==
  note: Berücksichtigung des temperaturabhängigen ohmschen Widerstands der Leitermaterialien in Rotor und Stator.
      | P_Verlust = (1+alpha*(T_aktuell - T_0))*P_Verlust_0
      | Dabei ist alpha der materialspezifische Temperaturkoeffizient des ohmschen Widerstandes.
      | P_Verlust_0 ist durch das Wirkungsgradkennfeld in "E-Maschine Verlustleistung" dargestellt. Dieses wurde für bestimmte Rotor und Stator-Temperaturen "T_Entwurf_*" berechnet. Diese Temperaturen dienen als Referenztemperaturen T_0.
  note: Aufteilung der ohmschen Wicklungsverluste innerhalb des Rotors auf die thermischen Massen Rotorstäbe (-nuten) & Kurzschlussring und innerhalb des Stators auf Wicklung in den Nuten & Wickelkopf.
  note: Aufteilung der ohmschen Wicklungsverluste auf Stator und Rotor nach konstanten Anteilen.
  T_EMaschine_SSL [K] : Inport
  T_EMaschine_WH [K] : Inport  Port=2
  T_EMaschine_ER [K] : Inport  Port=3
  T_EMaschine_RSL [K] : Inport  Port=4
  P_EMaschine_Verlust_Wicklung [W] : Inport  Port=5
  WirkZus-Verluste in Wicklung [W] : Inport  Port=6
  Add{,1..13} (14 alike) : Sum  Inputs=+-
  Bus Creator1 : BusCreator  Inputs=2
  Bus Creator2 : BusCreator  Inputs=2
  Bus Creator3 : BusCreator  Inputs=5
  Bus Creator4 : BusCreator  Inputs=5
  Bus Selector : BusSelector  OutputSignals=T_EMaschine_SSL_1 [K],T_EMaschine_SSL_2 [K],T_EMaschine_SSL_3 [K],T_EMaschine_SSL_4 [K],T_EMaschine_SSL_5 [K]
  Bus Selector1 : BusSelector  OutputSignals=T_EMaschine_WH_1 [K],T_EMaschine_WH_2 [K]
  Bus Selector2 : BusSelector  OutputSignals=T_EMaschine_ER_1 [K],T_EMaschine_ER_2 [K]
  Bus Selector3 : BusSelector  OutputSignals=T_EMaschine_RSL_1 [K],T_EMaschine_RSL_2 [K],T_EMaschine_RSL_3 [K],T_EMaschine_RSL_4 [K],T_EMaschine_RSL_5 [K]
  Constant : Constant  Value=T_Entwurf_Rotor
  Constant1 : Constant  Value=T_Entwurf_Stator
  Constant{2..15} (14 alike) : Constant
  Delay{1..14} (14 alike) : Delay
  Gain{,1,9..13} (7 alike) : Gain  Gain=alpha_Rotor
  Gain14 : Gain  Gain=1/2
  Gain15 : Gain  Gain=1/n_dis
  Gain{2..8} (7 alike) : Gain  Gain=alpha_Stator
  Product{1..14} (14 alike) : Product
  Share of stator winding in stator slot : Gain  Gain=m_SSL_L/(n_dis*m_SSL_L+2*m_WH_L)
  Share of stator winding in winding head : Gain  Gain=m_WH_L/(n_dis*m_SSL_L+2*m_WH_L)
  Sum{,1..14} (15 alike) : Sum  Inputs=|++
  Sum15 : Sum  Inputs=+++++
  Sum16 : Sum
  Sum17 : Sum
  Sum18 : Sum  Inputs=+++++
  share of rotor winding losses in end ring : Gain  Gain=Anteil_Rotor_Ringe
  share of rotor winding losses in rotor slot : Gain  Gain=1-Anteil_Rotor_Ringe
  share of winding losses in rotor : Gain  Gain=1-Anteil_Stator
  share of winding losses in stator : Gain  Gain=Anteil_Stator
  P_EMaschine_Verlust_SSL [W] : Outport
  P_EMaschine_Verlust_WH [W] : Outport  Port=2
  P_EMaschine_Verlust_ER [W] : Outport  Port=3
  P_EMaschine_Verlust_RSL [W] : Outport  Port=4
  P_EMaschine_Verlust_SSL_bus [W] : Outport  Port=5
  P_EMaschine_Verlust_WH_bus [W] : Outport  Port=6
  P_EMaschine_Verlust_ER_bus [W] : Outport  Port=7
  P_EMaschine_Verlust_RSL_bus [W] : Outport  Port=8
  wires:
  share of winding losses in stator/1 -> Share of stator winding in winding head/1, Share of stator winding in stator slot/1
  Sum/1 -> share of winding losses in stator/1, share of winding losses in rotor/1
  P_EMaschine_Verlust_Wicklung [W]/1 -> Sum/1
  WirkZus-Verluste in Wicklung [W]/1 -> Sum/2
  Constant1/1 -> Add7/2, Add6/2, Add5/2, Add4/2, Add3/2, Add2/2, Add8/2
  Add3/1 -> Delay2/1
  Add/1 -> Delay1/1
  Add1/1 -> Delay4/1
  Add2/1 -> Delay3/1
  Constant2/1 -> Sum1/2
  Constant3/1 -> Sum2/2
  Constant4/1 -> Sum3/2
  Constant5/1 -> Sum4/2
  Gain3/1 -> Sum4/1
  Gain2/1 -> Sum3/1
  Gain/1 -> Sum2/1
  Gain1/1 -> Sum1/1
  share of winding losses in rotor/1 -> share of rotor winding losses in end ring/1, share of rotor winding losses in rotor slot/1
  Share of stator winding in winding head/1 -> Product8/1, Product2/1
  Share of stator winding in stator slot/1 -> Product1/1, Product4/1, Product5/1, Product6/1, Product7/1
  Sum3/1 -> Product1/2
  Sum2/1 -> Product3/2
  Delay1/1 -> Gain1/1
  Delay4/1 -> Gain/1
  Delay3/1 -> Gain3/1
  Delay2/1 -> Gain2/1
  Add4/1 -> Delay5/1
  Gain4/1 -> Sum5/1
  Constant6/1 -> Sum5/2
  Delay5/1 -> Gain4/1
  Add5/1 -> Delay6/1
  Gain5/1 -> Sum6/1
  Constant7/1 -> Sum6/2
  Delay6/1 -> Gain5/1
  Add6/1 -> Delay7/1
  Gain6/1 -> Sum7/1
  Constant8/1 -> Sum7/2
  Delay7/1 -> Gain6/1
  Add7/1 -> Delay8/1
  Gain7/1 -> Sum8/1
  Constant9/1 -> Sum8/2
  Delay8/1 -> Gain7/1
  Bus Selector/2 -> Add4/1  "<T_EMaschine_SSL_2 [K]>"
  Bus Selector/3 -> Add5/1  "<T_EMaschine_SSL_3 [K]>"
  Bus Selector/4 -> Add6/1  "<T_EMaschine_SSL_4 [K]>"
  Sum8/1 -> Product7/2
  Sum7/1 -> Product6/2
  Sum6/1 -> Product5/2
  Sum5/1 -> Product4/2
  T_EMaschine_SSL [K]/1 -> Bus Selector/1
  Bus Selector/1 -> Add3/1  "<T_EMaschine_SSL_1 [K]>"
  Bus Selector/5 -> Add7/1  "<T_EMaschine_SSL_5 [K]>"
  T_EMaschine_WH [K]/1 -> Bus Selector1/1
  Add8/1 -> Delay9/1
  Delay9/1 -> Gain8/1
  Gain8/1 -> Sum9/1
  Constant10/1 -> Sum9/2
  Bus Selector1/1 -> Add8/1  "<T_EMaschine_WH_1 [K]>"
  Bus Selector1/2 -> Add2/1  "<T_EMaschine_WH_2 [K]>"
  Sum4/1 -> Product8/2
  Sum9/1 -> Product2/2
  Bus Selector2/1 -> Add1/1  "<T_EMaschine_ER_1 [K]>"
  T_EMaschine_ER [K]/1 -> Bus Selector2/1
  Sum10/1 -> Product9/2
  Delay10/1 -> Gain9/1
  Constant11/1 -> Sum10/2
  Gain9/1 -> Sum10/1
  Constant/1 -> Add13/2, Add12/2, Add11/2, Add10/2, Add9/2, Add1/2, Add/2
  Add9/1 -> Delay10/1
  Bus Selector2/2 -> Add9/1  "<T_EMaschine_ER_2 [K]>"
  Constant12/1 -> Sum11/2
  Delay11/1 -> Gain10/1
  Gain10/1 -> Sum11/1
  Add10/1 -> Delay11/1
  Add11/1 -> Delay12/1
  Delay12/1 -> Gain11/1
  Gain11/1 -> Sum12/1
  Constant13/1 -> Sum12/2
  Add12/1 -> Delay13/1
  Delay13/1 -> Gain12/1
  Gain12/1 -> Sum13/1
  Constant14/1 -> Sum13/2
  Add13/1 -> Delay14/1
  Delay14/1 -> Gain13/1
  Gain13/1 -> Sum14/1
  Constant15/1 -> Sum14/2
  T_EMaschine_RSL [K]/1 -> Bus Selector3/1
  Bus Selector3/1 -> Add13/1  "<T_EMaschine_RSL_1 [K]>"
  Bus Selector3/2 -> Add12/1  "<T_EMaschine_RSL_2 [K]>"
  Bus Selector3/3 -> Add11/1  "<T_EMaschine_RSL_3 [K]>"
  Bus Selector3/4 -> Add10/1  "<T_EMaschine_RSL_4 [K]>"
  Bus Selector3/5 -> Add/1  "<T_EMaschine_RSL_5 [K]>"
  Sum11/1 -> Product11/2
  Sum12/1 -> Product12/2
  Sum13/1 -> Product13/2
  Sum14/1 -> Product14/2
  Sum1/1 -> Product10/2
  Product14/1 -> Sum15/1, Bus Creator3/1  "P_EMaschine_Verlust_RSL_1 [W]"
  Product13/1 -> Sum15/2, Bus Creator3/2  "P_EMaschine_Verlust_RSL_2 [W]"
  Product12/1 -> Sum15/3, Bus Creator3/3  "P_EMaschine_Verlust_RSL_3 [W]"
  Product10/1 -> Sum15/5, Bus Creator3/5  "P_EMaschine_Verlust_RSL_5 [W]"
  Product11/1 -> Bus Creator3/4, Sum15/4  "P_EMaschine_Verlust_RSL_4 [W]"
  Sum15/1 -> P_EMaschine_Verlust_RSL [W]/1  "P_EMaschine_Verlust_RSL [W]"
  Bus Creator3/1 -> P_EMaschine_Verlust_RSL_bus [W]/1
  Product3/1 -> Sum16/1, Bus Creator1/1  "P_EMaschine_Verlust_ER_1 [W]"
  Product9/1 -> Bus Creator1/2, Sum16/2  "P_EMaschine_Verlust_ER_2 [W]"
  Bus Creator1/1 -> P_EMaschine_Verlust_ER_bus [W]/1
  Sum16/1 -> P_EMaschine_Verlust_ER [W]/1  "P_EMaschine_Verlust_ER [W]"
  Sum17/1 -> P_EMaschine_Verlust_WH [W]/1  "P_EMaschine_Verlust_WH [W]"
  Product2/1 -> Sum17/1, Bus Creator2/1  "P_EMaschine_Verlust_WH_1 [W]"
  Product8/1 -> Bus Creator2/2, Sum17/2  "P_EMaschine_Verlust_WH_2 [W]"
  Bus Creator2/1 -> P_EMaschine_Verlust_WH_bus [W]/1
  Product1/1 -> Sum18/1, Bus Creator4/1  "P_EMaschine_Verlust_SSL_1 [W]"
  Bus Creator4/1 -> P_EMaschine_Verlust_SSL_bus [W]/1
  Product5/1 -> Sum18/3, Bus Creator4/3  "P_EMaschine_Verlust_SSL_3 [W]"
  Product7/1 -> Sum18/5, Bus Creator4/5  "P_EMaschine_Verlust_SSL_5 [W]"
  Product4/1 -> Sum18/2, Bus Creator4/2  "P_EMaschine_Verlust_SSL_2 [W]"
  Product6/1 -> Bus Creator4/4, Sum18/4  "P_EMaschine_Verlust_SSL_4 [W]"
  Sum18/1 -> P_EMaschine_Verlust_SSL [W]/1  "P_EMaschine_Verlust_SSL [W]"
  share of rotor winding losses in rotor slot/1 -> Gain15/1
  share of rotor winding losses in end ring/1 -> Gain14/1
  Gain14/1 -> Product9/1, Product3/1
  Gain15/1 -> Product14/1, Product10/1, Product11/1, Product12/1, Product13/1

== system Antriebsstrangmodell_V1_4_n5/Antriebsstrang/E-Maschine Thermik/Thermisches Netzwerk/Subsystem ==

== system Antriebsstrangmodell_V1_4_n5/Antriebsstrang/E-Maschine Thermik/Thermisches Netzwerk/Subsystem1 ==

== system Antriebsstrangmodell_V1_4_n5/Antriebsstrang/E-Maschine Thermik/Wärmeübergangskoeffizienten Konvektion Luftspalt und Endcap-Luft/Endcap-Luft-Konvektion ==
  note: HTC_fconv stellt den Wärmeübergangs-
      | koeffizienten der erzwungen dar. Für diesen
      | wird bloß der geschwindigkeitsabhängige
      | Teil der empirischen Konvektions-Korrelation
      | der Innenluft genommen.
  note: Zusammenhang zwischen Geschwindigkeit der Innenluft und dem konvektiven Wärmeübergangskoeffizienten nach MELLOR 1991.
      | eta_IA ist hierbei der Lüfterwirkungsgrad, der das Verhältnis von Innenluftgeschwindigkeit zur Umfangsgeschwindigkeit des Kurzschlussrings am Rotor darstellt.
  n_EMaschine [min^-1] : Inport
  Add1 : Sum
  Constant1 : Constant  Value=0.29
  Constant2 : Constant
  Constant3 : Constant  Value=15.5
  Constant4 : Constant  Value=eta_IA
  Constant6 : Constant  Value=D_2r
  Divide1 : Product  Inputs=**
  Divide2 : Product  Inputs=**
  Divide3 : Product  Inputs=***
  Divide4 : Product  Inputs=**
  Gain : Gain  Gain=2*pi/60
  Gain1 : Gain  Gain=0.5
  HTC_Innenluft [W*m^-2*K^-1] : Outport
  HTC_fconv_Innenluft [W*m^-2*K^-1] : Outport  Port=2
  wires:
  Divide3/1 -> Divide1/1  "v_IA Innenluftgeschwindigkeit [m*s^-1]"
  n_EMaschine [min^-1]/1 -> Gain/1
  Constant6/1 -> Gain1/1
  Gain/1 -> Divide3/1
  Constant4/1 -> Divide3/2
  Gain1/1 -> Divide3/3
  Constant1/1 -> Divide1/2
  Divide1/1 -> Divide4/1, Add1/1
  Constant2/1 -> Add1/2
  Add1/1 -> Divide2/1
  Constant3/1 -> Divide4/2, Divide2/2
  Divide2/1 -> HTC_Innenluft [W*m^-2*K^-1]/1
  Divide4/1 -> HTC_fconv_Innenluft [W*m^-2*K^-1]/1
